simulink model "PID"  (R2022b)
settings: Solver=FixedStepAuto  StartTime=0.0  StopTime=time  FixedStep=0.01  RelTol=1e-3
undefined symbols (not defined in the file or in its folder): den, Kd_PID, Ki_PI, Ki_PID, Kp_P, Kp_PI, Kp_PID, num
settings Model: Creator=Xinrui  LastModifiedBy=Xinrui

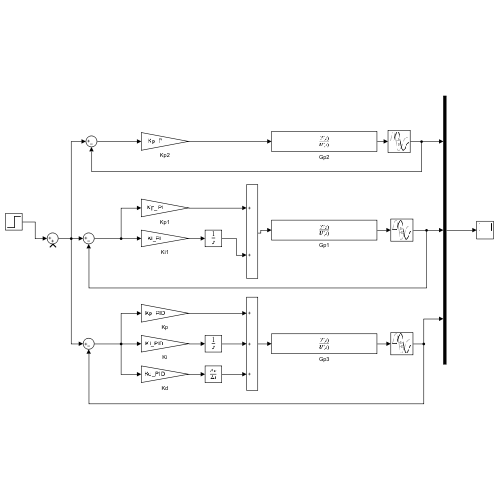
[thumbnail: Simulink's stored preview of the top-level diagram]
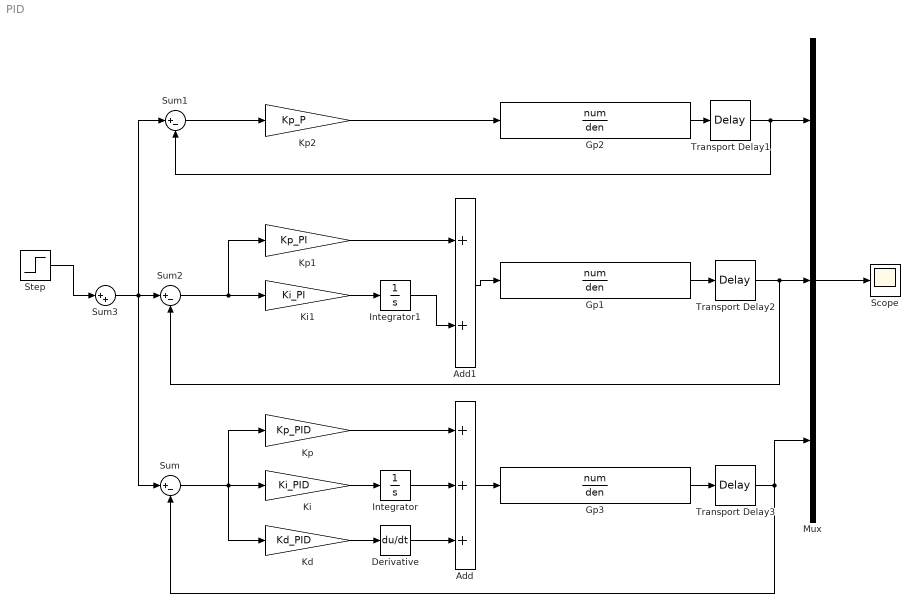
== system PID ==
  Add : Sum  Inputs=+++
  Add1 : Sum
  Derivative : Derivative
  Gp1 : TransferFcn  Numerator=num  Denominator=den
  Gp2 : TransferFcn  Numerator=num  Denominator=den
  Gp3 : TransferFcn  Numerator=num  Denominator=den
  Integrator : Integrator
  Integrator1 : Integrator
  Kd : Gain  Gain=Kd_PID
  Ki : Gain  Gain=Ki_PID
  Ki1 : Gain  Gain=Ki_PI
  Kp : Gain  Gain=Kp_PID
  Kp1 : Gain  Gain=Kp_PI
  Kp2 : Gain  Gain=Kp_P
  Mux : Mux  Inputs=3
  Scope : Scope
  Step : Step  SampleTime=0
  Sum : Sum  Inputs=|+-
  Sum1 : Sum  Inputs=|+-
  Sum2 : Sum  Inputs=|+-
  Sum3 : Sum  Inputs=|++
  Transport Delay1 : TransportDelay  DelayTime=t  BufferSize=2048
  Transport Delay2 : TransportDelay  DelayTime=t  BufferSize=2048
  Transport Delay3 : TransportDelay  DelayTime=t  BufferSize=2048
  wires:
  Sum/1 -> Kd/1, Kp/1, Ki/1
  Gp3/1 -> Transport Delay3/1
  Kp/1 -> Add/1
  Ki/1 -> Integrator/1
  Integrator/1 -> Add/2
  Add/1 -> Gp3/1
  Sum3/1 -> Sum1/1, Sum/1, Sum2/1
  Kd/1 -> Derivative/1
  Derivative/1 -> Add/3
  Mux/1 -> Scope/1
  Integrator1/1 -> Add1/2
  Sum2/1 -> Kp1/1, Ki1/1
  Ki1/1 -> Integrator1/1
  Kp1/1 -> Add1/1
  Add1/1 -> Gp1/1
  Gp1/1 -> Transport Delay2/1
  Kp2/1 -> Gp2/1
  Gp2/1 -> Transport Delay1/1
  Sum1/1 -> Kp2/1
  Transport Delay1/1 -> Mux/1, Sum1/2
  Transport Delay2/1 -> Mux/2, Sum2/2
  Transport Delay3/1 -> Mux/3, Sum/2
  Step/1 -> Sum3/1
